simulink model "verify_PipeBasic_mdl"  (R2013b)
settings: Solver=ode45  StartTime=0.0  StopTime=6*3600  MaxStep=600  RelTol=1e-3
libraries: carnot x4, simulink x1
settings Model: Creator=drhf  LastModifiedBy=drhf
settings DataIOCC: SignalLoggingSaveFormat=ModelDataLogs  SignalLogging=off
settings OptimizationCC: ExpressionDepthLimit=2147483647
settings DebuggingCC: FcnCallInpInsideContextMsg=UseLocalSettings  StateNameClashWarn=warning
settings GRTTargetCC: CombineOutputUpdateFcns=off  GRTInterface=on

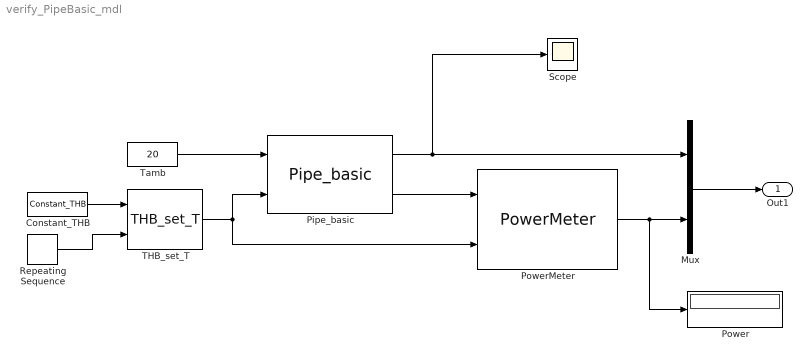
== system verify_PipeBasic_mdl ==
  Constant_THB : carnot/Source/Simple/Constant_THB  t=40  mdot=50/3600  p=1e5  mID=No Pressure Drop  fluid=Water  mix=0  mix2=0  mix3=0  dia=0.02  hgt=0
  Mux : Mux  Inputs=2
  Pipe_basic : carnot/Basic/Thermal_Models/Pipe_basic  vol="sqrt(0.01/(10*pi))      % 10 liter on 10 m"  L=10  uloss=1  effcond=0  cwall=0  t0=20  nodes=10
  Power : Display
  PowerMeter : carnot/Control/PowerMeter
  Repeating Sequence : simulink/Sources/Repeating Sequence  rep_seq_t=[0 1.99 2.01 3.99 4.01 7]*3600  rep_seq_y=[45 45 35 35 42 42]
  Scope : Scope
  THB_set_T : carnot/Source/Simple/THB_set_T
  Tamb : Constant  Value=20
  Out1 : Outport  SampleTime=600
  wires:
  Tamb/1 -> Pipe_basic/1
  THB_set_T/1 -> PowerMeter/2, Pipe_basic/2
  Mux/1 -> Out1/1
  PowerMeter/1 -> Power/1, Mux/2
  Pipe_basic/1 -> Scope/1, Mux/1
  Pipe_basic/2 -> PowerMeter/1
  Constant_THB/1 -> THB_set_T/1
  Repeating Sequence/1 -> THB_set_T/2
